simulink model "sampleModel1801"  (R2022a)
settings: Solver=FixedStepAuto  StartTime=0.0  StopTime=10.0  RelTol=1e-3
undefined symbols (not defined in the file): DiscIntNeverNeededParam, Newton, Raphson
libraries: simulink x66, slpidlib x17
(part 3 of 3)

== system sampleModel1801/cfblk47/cfblk11 ==
  cfblk1 : Inport
  cfblk14 : Inport  Port=2
  cfblk15 : Inport  Port=3
  cfblk10 : Sqrt  Operator=rSqrt  AlgorithmType=Newton-Raphson
  cfblk11 : Reshape
  cfblk12 : Reshape
  cfblk13 : Constant  Value=[-114160301.794608]  SampleTime=1
  cfblk16 : Delay  SampleTime=1
  cfblk3 : Delay  ShowEnablePort=on  SampleTime=1
      settings: InputPortMap=u0,e6
  cfblk4 : slpidlib/PID Controller (2DOF)  Controller=PID  Form=Parallel  TimeDomain=Discrete-time  UseExternalTs=off  SampleTime=1  IntegratorMethod=Forward Euler  FilterMethod=Forward Euler  ControllerParametersSource=internal  P=1  I=1  UseKiTs=off  D=0  N=100  UseFilter=on  b=1  c=1  TunerSelectOption=Transfer Function Based (PID Tuner App)  InitialConditionSource=internal  InitialConditionForIntegrator=0  InitialConditionForFilter=0  DifferentiatorICPrevScaledInput=0  ExternalReset=none  TrackingMode=off  Kt=1  LimitOutput=off  SatLimitsSource=internal  UpperSaturationLimit=inf  LowerSaturationLimit=-inf  LinearizeAsGain=off  AntiWindupMode=none  Kb=1  POutMin=[]  POutMax=[]  IOutMin=[]  IOutMax=[]  DOutMin=[]  DOutMax=[]  NOutMin=[]  NOutMax=[]  bOutMin=[]  bOutMax=[]  cOutMin=[]  cOutMax=[]  SumOutMin=[]  SumOutMax=[]  SaturationOutMin=[]  SaturationOutMax=[]  PParamMin=[]  PParamMax=[]  IParamMin=[]  IParamMax=[]  DParamMin=[]  DParamMax=[]  NParamMin=[]  NParamMax=[]  bParamMin=[]  bParamMax=[]  cParamMin=[]  cParamMax=[]  KbParamMin=[]  KbParamMax=[]  KtParamMin=[]  KtParamMax=[]  KbOutMin=[]  KbOutMax=[]  KtOutMin=[]  KtOutMax=[]  IntegratorOutMin=[]  IntegratorOutMax=[]  FilterOutMin=[]  FilterOutMax=[]  SumI1OutMin=[]  SumI1OutMax=[]  SumI2OutMin=[]  SumI2OutMax=[]  SumI3OutMin=[]  SumI3OutMax=[]  SumI4OutMin=[]  SumI4OutMax=[]  SumDOutMin=[]  SumDOutMax=[]  Sum1OutMin=[]  Sum1OutMax=[]  Sum2OutMin=[]  Sum2OutMax=[]  Sum3OutMin=[]  Sum3OutMax=[]  DifferentiatorOutMin=[]  DifferentiatorOutMax=[]  FilterDiffOutCoefMin=[]  FilterDiffOutCoefMax=[]  ReciprocalOutMin=[]  ReciprocalOutMax=[]  SumDenOutMin=[]  SumDenOutMax=[]  SumNumOutMin=[]  SumNumOutMax=[]  DivideOutMin=[]  DivideOutMax=[]  UdiffTsProdOutMin=[]  UdiffTsProdOutMax=[]  NTsProdOutMin=[]  NTsProdOutMax=[]  UintegralTsProdOutMin=[]  UintegralTsProdOutMax=[]  UngainTsProdOutMin=[]  UngainTsProdOutMax=[]  IntegratorContinuousStateAttributes=''  IntegratorStateMustResolveToSignalObject=off  IntegratorRTWStateStorageClass=Auto  FilterContinuousStateAttributes=''  FilterStateMustResolveToSignalObject=off  FilterRTWStateStorageClass=Auto  ParallelPVariant=InternalParameters  IdealPVariant=Disabled  IVariant=InternalParameters  DVariant=InternalParameters  bVariant=InternalParameters  cVariant=InternalParameters  IntegratorVariant=Discrete  SatVariant=Disabled  AWVariant=Passthrough  PCopyVariant=Disabled  TRVariant=Disabled  FdbkBlocksVariant=Forward  IdealPFdbkVariant=Disabled  SatFdbkVariant=Disabled  DerivativeFilterVariant=ForwardEulerFilter  NVariant=InternalParameters  NCopyVariant=Disabled  FilterICVariant=InternalICsFilter  IntegratorICVariant=InternalICs  ExternalResetVariant=Disabled  TRSumVariant=Passthrough  SumFdbkVariant=Disabled  SumVariant=Sum_PID  TsampFilterVariant=InternalTs  TsampNgainVariant=Passthrough  TsampIntegralVariant=Passthrough  ExternalSaturationOutDataTypeStr=Inherit: Same as second input
      settings: SourceProductBaseCode=SL
  cfblk5 : Reshape
  cfblk6 : DotProduct  OutDataTypeStr=Inherit: Inherit via internal rule
  cfblk7 : Sqrt
  cfblk8 : PermuteDimensions
  cfblk9 : Trigonometry
  cfblk2 : Outport
  wires:
  cfblk1/1 -> cfblk5/1
  cfblk9/1 -> cfblk7/1
  cfblk11/1 -> cfblk12/1
  cfblk15/1 -> cfblk3/1
  cfblk5/1 -> cfblk10/1
  cfblk4/1 -> cfblk6/1
  cfblk6/1 -> cfblk2/1
  cfblk8/1 -> cfblk11/1
  cfblk13/1 -> cfblk6/2
  cfblk3/1 -> cfblk8/1
  cfblk10/1 -> cfblk9/1
  cfblk7/1 -> cfblk4/1
  cfblk14/1 -> cfblk4/2
  cfblk12/1 -> cfblk16/1
  cfblk16/1 -> cfblk3/2

== system sampleModel1801/cfblk47/cfblk12 ==
  cfblk1 : Inport
  cfblk13 : Inport  Port=2
  cfblk10 : Bias  Bias=[569893462.336626]  SaturateOnIntegerOverflow=off
  cfblk11 : simulink/Math Operations/MinMax Running Resettable  Function=min  vinit=0.0
  cfblk12 : Constant  Value=[-214041770.452453]  SampleTime=1
  cfblk16 : Delay  SampleTime=1
  cfblk17 : Delay  SampleTime=1
  cfblk3 : Delay  ShowEnablePort=on  SampleTime=1
      settings: InputPortMap=u0,e6
  cfblk4 : DiscreteZeroPole  Poles=[0 0.5]  Gain=1
  cfblk5 : DiscreteFir  SampleTime=1
  cfblk6 : slpidlib/PID Controller  Controller=PID  Form=Parallel  TimeDomain=Discrete-time  UseExternalTs=off  SampleTime=1  IntegratorMethod=Forward Euler  FilterMethod=Forward Euler  ControllerParametersSource=internal  P=1  I=1  UseKiTs=off  D=0  N=100  UseFilter=on  TunerSelectOption=Transfer Function Based (PID Tuner App)  InitialConditionSource=internal  InitialConditionForIntegrator=0  InitialConditionForFilter=0  DifferentiatorICPrevScaledInput=0  ExternalReset=none  TrackingMode=off  Kt=1  LimitOutput=off  SatLimitsSource=internal  UpperSaturationLimit=inf  LowerSaturationLimit=-inf  LinearizeAsGain=off  AntiWindupMode=none  Kb=1  POutMin=[]  POutMax=[]  IOutMin=[]  IOutMax=[]  DOutMin=[]  DOutMax=[]  NOutMin=[]  NOutMax=[]  SumOutMin=[]  SumOutMax=[]  SaturationOutMin=[]  SaturationOutMax=[]  PParamMin=[]  PParamMax=[]  IParamMin=[]  IParamMax=[]  DParamMin=[]  DParamMax=[]  NParamMin=[]  NParamMax=[]  KbParamMin=[]  KbParamMax=[]  KtParamMin=[]  KtParamMax=[]  KbOutMin=[]  KbOutMax=[]  KtOutMin=[]  KtOutMax=[]  IntegratorOutMin=[]  IntegratorOutMax=[]  FilterOutMin=[]  FilterOutMax=[]  SumI1OutMin=[]  SumI1OutMax=[]  SumI2OutMin=[]  SumI2OutMax=[]  SumI3OutMin=[]  SumI3OutMax=[]  SumI4OutMin=[]  SumI4OutMax=[]  SumDOutMin=[]  SumDOutMax=[]  DifferentiatorOutMin=[]  DifferentiatorOutMax=[]  FilterDiffOutCoefMin=[]  FilterDiffOutCoefMax=[]  ReciprocalOutMin=[]  ReciprocalOutMax=[]  SumDenOutMin=[]  SumDenOutMax=[]  SumNumOutMin=[]  SumNumOutMax=[]  DivideOutMin=[]  DivideOutMax=[]  UdiffTsProdOutMin=[]  UdiffTsProdOutMax=[]  NTsProdOutMin=[]  NTsProdOutMax=[]  UintegralTsProdOutMin=[]  UintegralTsProdOutMax=[]  UngainTsProdOutMin=[]  UngainTsProdOutMax=[]  IntegratorContinuousStateAttributes=''  IntegratorStateMustResolveToSignalObject=off  IntegratorRTWStateStorageClass=Auto  FilterContinuousStateAttributes=''  FilterStateMustResolveToSignalObject=off  FilterRTWStateStorageClass=Auto  ParallelPVariant=InternalParameters  IdealPVariant=Disabled  IVariant=InternalParameters  DVariant=InternalParameters  IntegratorVariant=Discrete  SatVariant=Disabled  AWVariant=Passthrough  PCopyVariant=Disabled  TRVariant=Disabled  FdbkBlocksVariant=Forward  IdealPFdbkVariant=Disabled  SatFdbkVariant=Disabled  DerivativeFilterVariant=ForwardEulerFilter  NVariant=InternalParameters  NCopyVariant=Disabled  FilterICVariant=InternalICsFilter  IntegratorICVariant=InternalICs  ExternalResetVariant=Disabled  TRSumVariant=Passthrough  SumFdbkVariant=Disabled  SumVariant=Sum_PID  TsampFilterVariant=InternalTs  TsampNgainVariant=Passthrough  TsampIntegralVariant=Passthrough  ExternalSaturationOutDataTypeStr=Inherit: Same as second input  aMode=0
  cfblk7 : simulink/Discrete/Difference  ICPrevInput=0.0  OutMin=[]  OutMax=[]  OutDataTypeStr=Inherit: Inherit via back propagation  OutDataType=fixdt(1, 16)  OutScaling=2^-10  DoSatur=off
  cfblk8 : PermuteDimensions
  cfblk9 : Abs  SaturateOnIntegerOverflow=off
  cfblk2 : Outport
  cfblk14 : Outport  Port=2
  cfblk15 : Outport  Port=3
  wires:
  cfblk7/1 -> cfblk9/1
  cfblk11/1 -> cfblk4/1
  cfblk13/1 -> cfblk10/1
  cfblk8/1 -> cfblk14/1
  cfblk1/1 -> cfblk5/1
  cfblk10/1 -> cfblk2/1
  cfblk12/1 -> cfblk3/1, cfblk15/1
  cfblk6/1 -> cfblk8/1
  cfblk5/1 -> cfblk6/1, cfblk11/2
  cfblk4/1 -> cfblk3/2
  cfblk3/1 -> cfblk16/1
  cfblk16/1 -> cfblk11/1
  cfblk9/1 -> cfblk17/1
  cfblk17/1 -> cfblk7/1

== system sampleModel1801/cfblk47/cfblk13 ==
  cfblk1 : Inport
  cfblk9 : Inport  Port=2
  cfblk10 : Inport  Port=3
  cfblk13 : Delay  SampleTime=1
  cfblk14 : Delay  SampleTime=1
  cfblk3 : simulink/Discrete/Tapped Delay  vinit=0.0  samptime=-1  NumDelays=1  DelayOrder=Oldest  includeCurrent=off
  cfblk4 : DiscreteStateSpace
  cfblk5 : DiscreteTransferFcn  SampleTime=1
  cfblk6 : DiscreteFir  SampleTime=1
  cfblk7 : Sum  Inputs=+-
  cfblk8 : PermuteDimensions
  cfblk2 : Outport
  cfblk11 : Outport  Port=2
  cfblk12 : Outport  Port=3
  wires:
  cfblk3/1 -> cfblk7/1
  cfblk6/1 -> cfblk8/1
  cfblk10/1 -> cfblk11/1
  cfblk4/1 -> cfblk2/1
  cfblk1/1 -> cfblk4/1
  cfblk9/1 -> cfblk7/2
  cfblk7/1 -> cfblk12/1, cfblk5/1
  cfblk5/1 -> cfblk13/1
  cfblk13/1 -> cfblk3/1
  cfblk8/1 -> cfblk14/1
  cfblk14/1 -> cfblk6/1

== system sampleModel1801/cfblk47/cfblk14 ==
  cfblk1 : Inport
  cfblk10 : Inport  Port=2
  cfblk3 : Delay  SampleTime=1
  cfblk4 : DiscreteFilter  SampleTime=1
  cfblk5 : simulink/Discrete/Transfer Fcn Lead or Lag  PoleZ=0.95  ZeroZ=0.75  ICPrevOutput=0.0  ICPrevInput=0.0  DoSatur=off
      settings: SourceProductBaseCode=SL
  cfblk6 : Math  Operator=mod
  cfblk7 : Assignment  DiagnosticForDimensions=Warning  IndexOptions=Index vector (dialog)  Indices=1  OutputSizes=1
  cfblk8 : simulink/Math Operations/MinMax Running Resettable  Function=min  vinit=0.0
  cfblk9 : Constant  Value=[-397962416.782345]  SampleTime=1
  cfblk2 : Outport
  wires:
  cfblk3/1 -> cfblk8/1
  cfblk1/1 -> cfblk7/1, cfblk8/2
  cfblk4/1 -> cfblk2/1
  cfblk10/1 -> cfblk3/1
  cfblk5/1 -> cfblk4/1
  cfblk8/1 -> cfblk7/2
  cfblk7/1 -> cfblk6/1
  cfblk9/1 -> cfblk6/2
  cfblk6/1 -> cfblk5/1

== system sampleModel1801/cfblk47/cfblk15 ==
  cfblk1 : Inport
  cfblk9 : Inport  Port=2
  cfblk10 : Inport  Port=3
  cfblk11 : Inport  Port=4
  cfblk12 : Inport  Port=5
  cfblk14 : Delay  SampleTime=1
  cfblk3 : Reshape
  cfblk4 : Product  Inputs=**
  cfblk5 : Sum  Inputs=|++
  cfblk6 : Product  Inputs=**
  cfblk7 : Constant  Value=[928821836.448605]  SampleTime=1
  cfblk8 : Constant  Value=[-163429470.101786]  SampleTime=1
  cfblk2 : Outport
  cfblk13 : Outport  Port=2
  wires:
  cfblk10/1 -> cfblk6/1
  cfblk4/1 -> cfblk6/2
  cfblk1/1 -> cfblk4/2
  cfblk5/1 -> cfblk3/1
  cfblk3/1 -> cfblk13/1
  cfblk11/1 -> cfblk2/1
  cfblk12/1 -> cfblk5/1
  cfblk7/1 -> cfblk5/2
  cfblk6/1 -> cfblk14/1
  cfblk14/1 -> cfblk4/1

== system sampleModel1801/cfblk47/cfblk9 ==
  cfblk1 : Inport
  cfblk13 : Inport  Port=2
  cfblk10 : Constant  Value=[-738593309.628647]  SampleTime=1
  cfblk11 : Constant  Value=[-37136137.064962]  SampleTime=1
  cfblk12 : Constant  Value=[-699832431.659702]  SampleTime=1
  cfblk3 : DiscreteStateSpace
  cfblk4 : DiscreteZeroPole  Poles=[0 0.5]  Gain=1
  cfblk5 : simulink/Discrete/Difference  ICPrevInput=0.0  OutMin=[]  OutMax=[]  OutDataTypeStr=Inherit: Inherit via back propagation  OutDataType=fixdt(1, 16)  OutScaling=2^-10  DoSatur=off
  cfblk6 : Polyval  Coefs=[ +2.081618890e-019, -1.441693666e-014, +4.719686976e-010, -8.536869453e-006, +1.621573104e-001, -8.087801117e+001 ]
  cfblk7 : ComplexToRealImag
  cfblk8 : Sin  TimeSource=Use external signal  SampleTime=0
  cfblk9 : Abs  SaturateOnIntegerOverflow=off
  cfblk2 : Outport
  cfblk14 : Outport  Port=2
  wires:
  cfblk9/1 -> cfblk6/1
  cfblk11/1 -> cfblk5/1
  cfblk3/1 -> cfblk4/1
  cfblk13/1 -> cfblk8/1
  cfblk8/1 -> cfblk3/1
  cfblk5/1 -> cfblk9/1
  cfblk12/1 -> cfblk14/1
  cfblk1/1 -> cfblk7/1
  cfblk6/1 -> cfblk2/1

== system sampleModel1801/cfblk48/cfblk10 ==
  cfblk1 : Inport
  cfblk9 : Inport  Port=2
  cfblk3 : DiscreteIntegrator  ICPrevOutput=DiscIntNeverNeededParam  ICPrevScaledInput=DiscIntNeverNeededParam
  cfblk4 : DiscreteStateSpace
  cfblk5 : DiscreteFir  SampleTime=1
  cfblk6 : simulink/Math Operations/MinMax Running Resettable  Function=min  vinit=0.0
  cfblk7 : Sum  Inputs=+
  cfblk8 : Constant  Value=[-620440915.641846]  SampleTime=1
  cfblk2 : Outport
  cfblk10 : Outport  Port=2
  wires:
  cfblk9/1 -> cfblk10/1
  cfblk1/1 -> cfblk7/1
  cfblk8/1 -> cfblk4/1
  cfblk6/1 -> cfblk5/1
  cfblk5/1 -> cfblk3/1
  cfblk7/1 -> cfblk6/1
  cfblk3/1 -> cfblk2/1
  cfblk4/1 -> cfblk6/2

== system sampleModel1801/cfblk48/cfblk11 ==
  cfblk1 : Inport
  cfblk11 : Inport  Port=2
  cfblk12 : Inport  Port=3
  cfblk10 : Constant  Value=[714847942.188358]  SampleTime=1
  cfblk3 : Delay  DelayLengthSource=Input port  SampleTime=1
      settings: InputPortMap=u0,p1
  cfblk4 : DiscreteFir  SampleTime=1
  cfblk5 : Delay  ShowEnablePort=on  SampleTime=1
      settings: InputPortMap=u0,e6
  cfblk6 : Sum  Inputs=+
  cfblk7 : PermuteDimensions
  cfblk8 : Signum
  cfblk9 : Constant  Value=[-807249906.645020]  SampleTime=1
  cfblk2 : Outport
  wires:
  cfblk6/1 -> cfblk8/1
  cfblk4/1 -> cfblk7/1
  cfblk5/1 -> cfblk2/1
  cfblk7/1 -> cfblk6/1
  cfblk11/1 -> cfblk5/1
  cfblk10/1 -> cfblk3/1
  cfblk12/1 -> cfblk5/2
  cfblk1/1 -> cfblk4/1
  cfblk8/1 -> cfblk3/2

== system sampleModel1801/cfblk50/cfblk11 ==
  cfblk1 : Inport
  Action Port : ActionPort  ActionPortLabel=if(u1 >= 0)
  cfblk3 : DiscreteFilter
  cfblk4 : simulink/Discrete/Tapped Delay  vinit=0.0  samptime=-1  NumDelays=1  DelayOrder=Oldest  includeCurrent=off
  cfblk5 : simulink/Discrete/Difference  ICPrevInput=0.0  OutMin=[]  OutMax=[]  OutDataTypeStr=Inherit: Inherit via back propagation  OutDataType=fixdt(1, 16)  OutScaling=2^-10  DoSatur=off
  cfblk6 : UnaryMinus
  cfblk7 : Sqrt
  cfblk8 : Delay
  cfblk2 : Outport
  wires:
  cfblk6/1 -> cfblk2/1
  cfblk3/1 -> cfblk5/1
  cfblk5/1 -> cfblk7/1
  cfblk7/1 -> cfblk4/1
  cfblk1/1 -> cfblk6/1
  cfblk4/1 -> cfblk8/1
  cfblk8/1 -> cfblk3/1

== system sampleModel1801/cfblk50/cfblk12 ==
  cfblk1 : Inport
  cfblk7 : Inport  Port=2
  cfblk8 : Inport  Port=3
  Action Port : ActionPort  ActionPortLabel=else
  cfblk3 : simulink/Discrete/Difference  ICPrevInput=0.0  OutMin=[]  OutMax=[]  OutDataTypeStr=Inherit: Inherit via back propagation  OutDataType=fixdt(1, 16)  OutScaling=2^-10  DoSatur=off
  cfblk4 : DiscreteFir
  cfblk5 : Constant  Value=[772950897.844507]  SampleTime=1
  cfblk6 : Constant  Value=[-205223902.750779]  SampleTime=1
  cfblk2 : Outport
  wires:
  cfblk5/1 -> cfblk3/1
  cfblk3/1 -> cfblk4/1
  cfblk4/1 -> cfblk2/1

== system sampleModel1801/cfblk50/cfblk6 ==
  cfblk1 : Inport
  cfblk8 : Inport  Port=2
  cfblk9 : Inport  Port=3
  cfblk3 : DotProduct  OutDataTypeStr=Inherit: Inherit via internal rule
  cfblk4 : Sin  TimeSource=Use external signal  SampleTime=0
  cfblk5 : Squeeze
  cfblk6 : Sin  TimeSource=Use external signal  SampleTime=0
  cfblk7 : Sum  Inputs=+
  cfblk2 : Outport
  wires:
  cfblk1/1 -> cfblk2/1
  cfblk8/1 -> cfblk4/1
  cfblk4/1 -> cfblk7/1
  cfblk6/1 -> cfblk3/1
  cfblk9/1 -> cfblk6/1
  cfblk7/1 -> cfblk5/1
  cfblk5/1 -> cfblk3/2

== system sampleModel1801/cfblk51/cfblk5 ==
  cfblk1 : Inport
  cfblk11 : Inport  Port=2
  cfblk12 : Inport  Port=3
  cfblk13 : Inport  Port=4
  cfblk10 : Constant  Value=[-101288820.565528]  SampleTime=1
  cfblk3 : simulink/Discrete/Difference  ICPrevInput=0.0  OutMin=[]  OutMax=[]  OutDataTypeStr=Inherit: Inherit via back propagation  OutDataType=fixdt(1, 16)  OutScaling=2^-10  DoSatur=off
  cfblk4 : Delay
  cfblk5 : ComplexToMagnitudeAngle
  cfblk6 : Product  Inputs=**
  cfblk7 : Trigonometry
  cfblk8 : Signum
  cfblk9 : Constant  Value=[-983696434.415174]  SampleTime=1
  cfblk2 : Outport
  cfblk14 : Outport  Port=2
  wires:
  cfblk4/1 -> cfblk8/1
  cfblk10/1 -> cfblk5/1
  cfblk13/1 -> cfblk3/1
  cfblk9/1 -> cfblk4/1
  cfblk11/1 -> cfblk6/1
  cfblk1/1 -> cfblk6/2
  cfblk7/1 -> cfblk2/1
  cfblk12/1 -> cfblk7/1
  cfblk5/1 -> cfblk14/1
